simulink model "ARC_DTm"  (R2025b)
settings: Solver=FixedStepAuto  StartTime=0.0  StopTime=10080  FixedStep=1  RelTol=1e-3
PreLoadFcn:
  | %For Preload, set the working path
  | modelFolder = fileparts(which(bdroot));
  | addpath(genpath(modelFolder));
StartFcn:
  | tic
StopFcn:
  | fprintf("Sim Time: %.02f min", toc/60)
values from neighbouring files (symbols this model uses):
  batteryScenario = p.batteryScenario    [RUNSIM_ParameterSweep.m]    (also in _RUNSIM_ParameterSweep.m)
  Electricity_SalePriceModifier = 50/100    (= 0.5)    [RUNSIM_ParameterSweep.m]    (also in _RUNSIM_ParameterSweep.m)
  LUT = LUT_load.gamLUT    [RUNSIM_ParameterSweep.m]    (also in _RUNSIM_ParameterSweep.m)
  minimum_UF_system_flow = 5833    [RUNSIM_ParameterSweep.m]    (also in _RUNSIM_ParameterSweep.m)
  PROS1_recoveryrate = 61    [RUNSIM_ParameterSweep.m]    (also in _RUNSIM_ParameterSweep.m)
  PROS2_recoveryrate = 62    [RUNSIM_ParameterSweep.m]    (also in _RUNSIM_ParameterSweep.m)
  ROstabilization_time = p.ROstabilization_time    [RUNSIM_ParameterSweep.m]    (also in _RUNSIM_ParameterSweep.m)
  solarModifier = maximum_solar_generation / 300    [RUNSIM_ParameterSweep.m]    (also in _RUNSIM_ParameterSweep.m)
  TSRO_recoveryrate = 51    [RUNSIM_ParameterSweep.m]    (also in _RUNSIM_ParameterSweep.m)
  UF_RecoveryRate = 96    [RUNSIM_ParameterSweep.m]    (also in _RUNSIM_ParameterSweep.m)
undefined symbols (not defined in the file or in its folder): A_PROS1, A_PROS2, A_TSRO, B_PROS1, B_PROS2, B_TSRO, BW_Max_Time, BW_Max_Vol_gal, CEB_Max_Time, CEB_Max_Vol_gal, CIP_Max_Time, E, FF, h, L, w
libraries: simulink x40
(part 6 of 11)

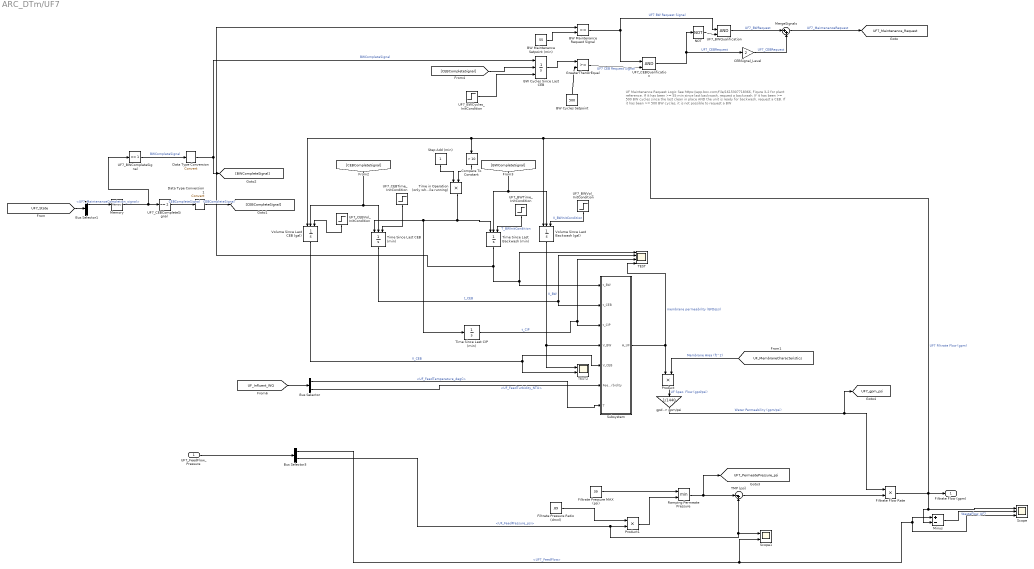
== system ARC_DTm/UF7 ==
  note: UF Maintenance Request Logic
      | See https://app.box.com/file/1615307718366, Figure 3-2 for plant reference.
      |
      | If it has been >= 55 min since last backwash, request a backwash.
      | If it has been >= 500 BW cycles since the last clean in place AND the unit is ready for backwash, request a CEB.
      | If it has been >= 500 BW cycles, it is not possible to request a BW
  UF7_FeedFlow_Pressure : Inport
  BW Cycles Setpoint : Constant  Value=500
  BW Cycles Since Last CEB : Integrator  ExternalReset=rising  InitialConditionSource=external  InitialCondition=5
  BW Maintenance Request Signal : RelationalOperator  OutDataTypeStr=boolean  RndMeth=Simplest  InputSameDT=off
  BW Maintenance Setpoint (min) : Constant  Value=55
  Bus Selector : BusSelector  OutputSignals=UF_FeedTemperature_degC,UF_FeedTurbidity_NTU
  Bus Selector1 : BusSelector  OutputSignals=UF7_MaintenanceCompletion_signal,UF7_OperationsState_signal
  Bus Selector3 : BusSelector  OutputSignals=UF7_FeedFlow,UF_FeedPressure_psi
  CEBSignal_Level : Gain  Gain=2  OutDataTypeStr=double
  Compare To Constant : simulink/Logic and Bit Operations/Compare To Constant  relop=>  const=10  OutDataTypeStr=boolean
  Data Type Conversion : DataTypeConversion  SaturateOnIntegerOverflow=off  RndMeth=Floor
  Data Type Conversion1 : DataTypeConversion  SaturateOnIntegerOverflow=off  RndMeth=Floor
  Filtrate Flow Rate : Product
  Filtrate Pressure MAX (psi) : Constant  Value=39
  Filtrate Pressure Ratio (dmnl) : Constant  Value=.89
  GreaterThanOrEqual : RelationalOperator  OutDataTypeStr=boolean  RndMeth=Simplest  InputSameDT=off
  Memory : Memory
  MergeSignals : Sum  Inputs=|++
  Minus : Sum  Inputs=+-
  NOT : Logic  Operator=NOT  IconShape=distinctive  AllPortsSameDT=off  OutDataTypeStr=boolean
  Product : Product
  Product1 : Product
  Ramping Permeate Pressure : MinMax  Inputs=2
  Scope : Scope  NumInputPorts=3
      settings: ActiveDisplayYMinimum=-126.71796384165732  ActiveDisplayYMaximum=1140.4616745749161  DataLoggingVariableName=ScopeData10
  Scope1 : Scope  NumInputPorts=2
      settings: ActiveDisplayYMinimum=-129.2228584451866  ActiveDisplayYMaximum=1163.0057260066797  DataLoggingVariableName=ScopeData11
  Step Add (min) : Constant
  Subsystem : Subsystem
  TEST : Scope  NumInputPorts=4
      settings: ActiveDisplayYMinimum=13.625  ActiveDisplayYMaximum=27.375  DataLoggingVariableName=ScopeData3
  TEST2 : Scope  NumInputPorts=2
      settings: ActiveDisplayYMinimum=-311929.86683332996  ActiveDisplayYMaximum=2.8073688014999703E+6  DataLoggingVariableName=ScopeData4
  TMP (psi) : Sum  Inputs=|-+
  Time Since Last Backwash (min) : Integrator  ExternalReset=level hold  InitialConditionSource=external  InitialCondition=26
  Time Since Last CEB (min) : Integrator  ExternalReset=level hold  InitialConditionSource=external  InitialCondition=4833
  Time Since Last CIP (min) : Integrator  InitialCondition=round(CIP_Max_Time*rand())
  Time in Operation (only while running) : Product
  UF7_BWCompleteSignal : simulink/Logic and Bit Operations/Compare To Constant  relop===  const=1  OutDataTypeStr=uint8
  UF7_BWCycles_InitCondition : Step  Before=round(500 * rand())  After=0  SampleTime=0
  UF7_BWQualification : Logic  IconShape=distinctive  AllPortsSameDT=off  OutDataTypeStr=boolean
  UF7_BWTime_InitCondition : Step  Before=round(BW_Max_Time*rand())  After=0  SampleTime=0
  UF7_BWVol_InitCondition : Step  Before=round(BW_Max_Vol_gal*rand())  After=0  SampleTime=0
  UF7_CEBCompleteSignal : simulink/Logic and Bit Operations/Compare To Constant  relop===  const=2  OutDataTypeStr=uint8
  UF7_CEBQualification : Logic  IconShape=distinctive  AllPortsSameDT=off  OutDataTypeStr=boolean
  UF7_CEBTime_InitCondition : Step  Before=round(CEB_Max_Time*rand())  After=0  SampleTime=0
  UF7_CEBVol_InitCondition : Step  Before=round(CEB_Max_Vol_gal*rand())  After=0  SampleTime=0
  Volume Since Last Backwash (gal) : Integrator  ExternalReset=level hold  InitialConditionSource=external  InitialCondition=34330
  Volume Since Last CEB (gal) : Integrator  ExternalReset=rising  InitialConditionSource=external  InitialCondition=2777254
  "gpd -> gpm/psi" : Gain  Gain=1/1440
  Filtrate Flow (gpm) : Outport
  tag scope: UF7_Maintenance_Request=global, UF7_PermeatePressure_psi=global, UF7_gpm_psi=global
  wires:
  Volume Since Last Backwash (gal)/1 -> Subsystem/4(V_BW), TEST2/1  "V_BW"
  Time Since Last Backwash (min)/1 -> BW Maintenance Request Signal/1, Subsystem/1(t_BW), TEST/1
  Product/1 -> "gpd -> gpm/psi"/1  "UF Spec. Flow (gpd/psi)"
  [UF_MembraneCharacteristics] -> Product/2  "Membrane Area (ft^2)"
  "gpd -> gpm/psi"/1 -> Filtrate Flow Rate/1, [UF7_gpm_psi]  "Water Permeability (gpm/psi)"
  Time in Operation (only while running)/1 -> Time Since Last Backwash (min)/1, Time Since Last CEB (min)/1, Time Since Last CIP (min)/1
  Filtrate Flow Rate/1 -> Scope/1, Minus/2, Volume Since Last Backwash (gal)/1, Volume Since Last CEB (gal)/1, Compare To Constant/1, Filtrate Flow (gpm)/1  "UF7 Filtrate Flow (gpm)"
  Time Since Last CEB (min)/1 -> Subsystem/2(t_CEB), TEST/2  "t_CEB"
  Volume Since Last CEB (gal)/1 -> Subsystem/5(V_CEB), TEST2/2  "V_CEB"
  Time Since Last CIP (min)/1 -> Subsystem/3(t_CIP), TEST/3  "t_CIP"
  Filtrate Pressure MAX (psi)/1 -> Ramping Permeate Pressure/1
  [UF_Influent_WQ] -> Bus Selector/1
  Bus Selector/1 -> Subsystem/7(T)  "<UF_FeedTemperature_degC>"
  UF7_FeedFlow_Pressure/1 -> Bus Selector3/1
  Filtrate Pressure Ratio (dmnl)/1 -> Product1/1
  Product1/1 -> Ramping Permeate Pressure/2
  Ramping Permeate Pressure/1 -> [UF7_PermeatePressure_psi], TMP (psi)/1
  TMP (psi)/1 -> Filtrate Flow Rate/2
  BW Maintenance Setpoint (min)/1 -> BW Maintenance Request Signal/2
  BW Cycles Since Last CEB/1 -> GreaterThanOrEqual/1
  BW Cycles Setpoint/1 -> GreaterThanOrEqual/2
  Bus Selector/2 -> Subsystem/6(Feed Turbidity)  "<UF_FeedTurbidity_NTU>"
  [UF7_State] -> Bus Selector1/1
  MergeSignals/1 -> [UF7_Maintenance_Request]  "UF7_MaintenanceRequest"
  UF7_CEBCompleteSignal/1 -> Data Type Conversion1/1  "CEBCompleteSignal"
  [CEBCompleteSignal] -> Volume Since Last CEB (gal)/2, Time Since Last CEB (min)/2
  Data Type Conversion/1 -> [BWCompleteSignal], BW Cycles Since Last CEB/1  "BWCompleteSignal"
  [BWCompleteSignal] -> Volume Since Last Backwash (gal)/2, Time Since Last Backwash (min)/2
  [CEBCompleteSignal] -> BW Cycles Since Last CEB/2
  Bus Selector1/1 -> Memory/1  "<UF7_MaintenanceCompletion_signal>"
  UF7_BWCompleteSignal/1 -> Data Type Conversion/1  "BWCompleteSignal"
  Data Type Conversion1/1 -> [CEBCompleteSignal]  "CEBCompleteSignal"
  UF7_BWCycles_InitCondition/1 -> BW Cycles Since Last CEB/3
  Subsystem/1(A_UF) -> TEST/4, Product/1  "membrane permeability (GFD/psi)"
  UF7_BWTime_InitCondition/1 -> Time Since Last Backwash (min)/3  "T_BWInitCondition"
  UF7_CEBVol_InitCondition/1 -> Volume Since Last CEB (gal)/3
  UF7_CEBTime_InitCondition/1 -> Time Since Last CEB (min)/3
  UF7_BWVol_InitCondition/1 -> Volume Since Last Backwash (gal)/3  "V_BWInitCondition"
  Step Add (min)/1 -> Time in Operation (only while running)/1
  Compare To Constant/1 -> Time in Operation (only while running)/2
  Memory/1 -> UF7_BWCompleteSignal/1, UF7_CEBCompleteSignal/1
  UF7_BWQualification/1 -> MergeSignals/1  "UF7_BWRequest"
  GreaterThanOrEqual/1 -> UF7_CEBQualification/2  "UF7 CEB Request Signal"
  UF7_CEBQualification/1 -> CEBSignal_Level/1, NOT/1  "UF7_CEBRequest"
  BW Maintenance Request Signal/1 -> UF7_BWQualification/1, UF7_CEBQualification/1  "UF7 BW Request Signal"
  NOT/1 -> UF7_BWQualification/2
  CEBSignal_Level/1 -> MergeSignals/2  "UF7_CEBRequest"
  Bus Selector3/1 -> Scope1/2, Minus/1, Scope/3  "<UF7_FeedFlow>"
  Bus Selector3/2 -> TMP (psi)/2, Scope1/1, Product1/2  "<UF_FeedPressure_psi>"
  Minus/1 -> Scope/2  "WasteFlow_UF7"

== system ARC_DTm/UF8 ==
  note: UF Maintenance Request Logic
      | See https://app.box.com/file/1615307718366, Figure 3-2 for plant reference.
      |
      | If it has been >= 55 min since last backwash, request a backwash.
      | If it has been >= 500 BW cycles since the last clean in place AND the unit is ready for backwash, request a CEB.
      | If it has been >= 500 BW cycles, it is not possible to request a BW
  UF8_FeedFlow_Pressure : Inport
  BW Cycles Setpoint : Constant  Value=500
  BW Cycles Since Last CEB : Integrator  ExternalReset=rising  InitialConditionSource=external  InitialCondition=5
  BW Maintenance Request Signal : RelationalOperator  OutDataTypeStr=boolean  RndMeth=Simplest  InputSameDT=off
  BW Maintenance Setpoint (min) : Constant  Value=55
  Bus Selector : BusSelector  OutputSignals=UF_FeedTemperature_degC,UF_FeedTurbidity_NTU
  Bus Selector1 : BusSelector  OutputSignals=UF8_MaintenanceCompletion_signal,UF8_OperationsState_signal
  Bus Selector3 : BusSelector  OutputSignals=UF8_FeedFlow,UF_FeedPressure_psi
  CEBSignal_Level : Gain  Gain=2  OutDataTypeStr=double
  Compare To Constant : simulink/Logic and Bit Operations/Compare To Constant  relop=>  const=10  OutDataTypeStr=boolean
  Data Type Conversion : DataTypeConversion  SaturateOnIntegerOverflow=off  RndMeth=Floor
  Data Type Conversion1 : DataTypeConversion  SaturateOnIntegerOverflow=off  RndMeth=Floor
  Filtrate Flow Rate : Product
  Filtrate Pressure MAX (psi) : Constant  Value=39
  Filtrate Pressure Ratio (dmnl) : Constant  Value=.89
  GreaterThanOrEqual : RelationalOperator  OutDataTypeStr=boolean  RndMeth=Simplest  InputSameDT=off
  Memory : Memory
  MergeSignals : Sum  Inputs=|++
  Minus : Sum  Inputs=+-
  NOT : Logic  Operator=NOT  IconShape=distinctive  AllPortsSameDT=off  OutDataTypeStr=boolean
  Product : Product
  Product1 : Product
  Ramping Permeate Pressure : MinMax  Inputs=2
  Scope : Scope  NumInputPorts=3
      settings: ActiveDisplayYMinimum=-126.71796384165732  ActiveDisplayYMaximum=1140.4616745749161  DataLoggingVariableName=ScopeData10
  Scope1 : Scope  NumInputPorts=2
      settings: ActiveDisplayYMinimum=-129.2228584451866  ActiveDisplayYMaximum=1163.0057260066797  DataLoggingVariableName=ScopeData11
  Step Add (min) : Constant
  Subsystem : Subsystem
  TEST : Scope  NumInputPorts=4
      settings: ActiveDisplayYMinimum=13.625  ActiveDisplayYMaximum=27.375  DataLoggingVariableName=ScopeData3
  TEST2 : Scope  NumInputPorts=2
      settings: ActiveDisplayYMinimum=-311929.86683332996  ActiveDisplayYMaximum=2.8073688014999703E+6  DataLoggingVariableName=ScopeData4
  TMP (psi) : Sum  Inputs=|-+
  Time Since Last Backwash (min) : Integrator  ExternalReset=level hold  InitialConditionSource=external  InitialCondition=26
  Time Since Last CEB (min) : Integrator  ExternalReset=level hold  InitialConditionSource=external  InitialCondition=4833
  Time Since Last CIP (min) : Integrator  InitialCondition=round(CIP_Max_Time*rand())
  Time in Operation (only while running) : Product
  UF8_BWCompleteSignal : simulink/Logic and Bit Operations/Compare To Constant  relop===  const=1  OutDataTypeStr=uint8
  UF8_BWCycles_InitCondition : Step  Before=round(500 * rand())  After=0  SampleTime=0
  UF8_BWQualification : Logic  IconShape=distinctive  AllPortsSameDT=off  OutDataTypeStr=boolean
  UF8_BWTime_InitCondition : Step  Before=round(BW_Max_Time*rand())  After=0  SampleTime=0
  UF8_BWVol_InitCondition : Step  Before=round(BW_Max_Vol_gal*rand())  After=0  SampleTime=0
  UF8_CEBCompleteSignal : simulink/Logic and Bit Operations/Compare To Constant  relop===  const=2  OutDataTypeStr=uint8
  UF8_CEBQualification : Logic  IconShape=distinctive  AllPortsSameDT=off  OutDataTypeStr=boolean
  UF8_CEBTime_InitCondition : Step  Before=round(CEB_Max_Time*rand())  After=0  SampleTime=0
  UF8_CEBVol_InitCondition : Step  Before=round(CEB_Max_Vol_gal*rand())  After=0  SampleTime=0
  Volume Since Last Backwash (gal) : Integrator  ExternalReset=level hold  InitialConditionSource=external  InitialCondition=34330
  Volume Since Last CEB (gal) : Integrator  ExternalReset=rising  InitialConditionSource=external  InitialCondition=2777254
  "gpd -> gpm/psi" : Gain  Gain=1/1440
  Filtrate Flow (gpm) : Outport
  tag scope: UF8_Maintenance_Request=global, UF8_PermeatePressure_psi=global, UF8_gpm_psi=global
  wires:
  Volume Since Last Backwash (gal)/1 -> Subsystem/4(V_BW), TEST2/1  "V_BW"
  Time Since Last Backwash (min)/1 -> BW Maintenance Request Signal/1, Subsystem/1(t_BW), TEST/1
  Product/1 -> "gpd -> gpm/psi"/1  "UF Spec. Flow (gpd/psi)"
  [UF_MembraneCharacteristics] -> Product/2  "Membrane Area (ft^2)"
  "gpd -> gpm/psi"/1 -> Filtrate Flow Rate/1, [UF8_gpm_psi]  "Water Permeability (gpm/psi)"
  Time in Operation (only while running)/1 -> Time Since Last Backwash (min)/1, Time Since Last CEB (min)/1, Time Since Last CIP (min)/1
  Filtrate Flow Rate/1 -> Scope/1, Minus/2, Volume Since Last Backwash (gal)/1, Volume Since Last CEB (gal)/1, Compare To Constant/1, Filtrate Flow (gpm)/1  "UF8 Filtrate Flow (gpm)"
  Time Since Last CEB (min)/1 -> Subsystem/2(t_CEB), TEST/2  "t_CEB"
  Volume Since Last CEB (gal)/1 -> Subsystem/5(V_CEB), TEST2/2  "V_CEB"
  Time Since Last CIP (min)/1 -> Subsystem/3(t_CIP), TEST/3  "t_CIP"
  Filtrate Pressure MAX (psi)/1 -> Ramping Permeate Pressure/1
  [UF_Influent_WQ] -> Bus Selector/1
  Bus Selector/1 -> Subsystem/7(T)  "<UF_FeedTemperature_degC>"
  UF8_FeedFlow_Pressure/1 -> Bus Selector3/1
  Filtrate Pressure Ratio (dmnl)/1 -> Product1/1
  Product1/1 -> Ramping Permeate Pressure/2
  Ramping Permeate Pressure/1 -> [UF8_PermeatePressure_psi], TMP (psi)/1
  TMP (psi)/1 -> Filtrate Flow Rate/2
  BW Maintenance Setpoint (min)/1 -> BW Maintenance Request Signal/2
  BW Cycles Since Last CEB/1 -> GreaterThanOrEqual/1
  BW Cycles Setpoint/1 -> GreaterThanOrEqual/2
  Bus Selector/2 -> Subsystem/6(Feed Turbidity)  "<UF_FeedTurbidity_NTU>"
  [UF8_State] -> Bus Selector1/1
  MergeSignals/1 -> [UF8_Maintenance_Request]  "UF8_MaintenanceRequest"
  UF8_CEBCompleteSignal/1 -> Data Type Conversion1/1  "CEBCompleteSignal"
  [CEBCompleteSignal] -> Volume Since Last CEB (gal)/2, Time Since Last CEB (min)/2
  Data Type Conversion/1 -> [BWCompleteSignal], BW Cycles Since Last CEB/1  "BWCompleteSignal"
  [BWCompleteSignal] -> Volume Since Last Backwash (gal)/2, Time Since Last Backwash (min)/2
  [CEBCompleteSignal] -> BW Cycles Since Last CEB/2
  Bus Selector1/1 -> Memory/1  "<UF8_MaintenanceCompletion_signal>"
  UF8_BWCompleteSignal/1 -> Data Type Conversion/1  "BWCompleteSignal"
  Data Type Conversion1/1 -> [CEBCompleteSignal]  "CEBCompleteSignal"
  UF8_BWCycles_InitCondition/1 -> BW Cycles Since Last CEB/3
  Subsystem/1(A_UF) -> TEST/4, Product/1  "membrane permeability (GFD/psi)"
  UF8_BWTime_InitCondition/1 -> Time Since Last Backwash (min)/3  "T_BWInitCondition"
  UF8_CEBVol_InitCondition/1 -> Volume Since Last CEB (gal)/3
  UF8_CEBTime_InitCondition/1 -> Time Since Last CEB (min)/3
  UF8_BWVol_InitCondition/1 -> Volume Since Last Backwash (gal)/3  "V_BWInitCondition"
  Step Add (min)/1 -> Time in Operation (only while running)/1
  Compare To Constant/1 -> Time in Operation (only while running)/2
  Memory/1 -> UF8_BWCompleteSignal/1, UF8_CEBCompleteSignal/1
  UF8_BWQualification/1 -> MergeSignals/1  "UF8_BWRequest"
  GreaterThanOrEqual/1 -> UF8_CEBQualification/2  "UF8 CEB Request Signal"
  UF8_CEBQualification/1 -> CEBSignal_Level/1, NOT/1  "UF8_CEBRequest"
  BW Maintenance Request Signal/1 -> UF8_BWQualification/1, UF8_CEBQualification/1  "UF8 BW Request Signal"
  NOT/1 -> UF8_BWQualification/2
  CEBSignal_Level/1 -> MergeSignals/2  "UF8_CEBRequest"
  Bus Selector3/1 -> Scope1/2, Minus/1, Scope/3  "<UF8_FeedFlow>"
  Bus Selector3/2 -> TMP (psi)/2, Scope1/1, Product1/2  "<UF_FeedPressure_psi>"
  Minus/1 -> Scope/2  "WasteFlow_UF8"

== system ARC_DTm/UF9 ==
  note: UF Maintenance Request Logic
      | See https://app.box.com/file/1615307718366, Figure 3-2 for plant reference.
      |
      | If it has been >= 55 min since last backwash, request a backwash.
      | If it has been >= 500 BW cycles since the last clean in place AND the unit is ready for backwash, request a CEB.
      | If it has been >= 500 BW cycles, it is not possible to request a BW
  UF9_FeedFlow_Pressure : Inport
  BW Cycles Setpoint : Constant  Value=500
  BW Cycles Since Last CEB : Integrator  ExternalReset=rising  InitialConditionSource=external  InitialCondition=5
  BW Maintenance Request Signal : RelationalOperator  OutDataTypeStr=boolean  RndMeth=Simplest  InputSameDT=off
  BW Maintenance Setpoint (min) : Constant  Value=55
  Bus Selector : BusSelector  OutputSignals=UF_FeedTemperature_degC,UF_FeedTurbidity_NTU
  Bus Selector1 : BusSelector  OutputSignals=UF9_MaintenanceCompletion_signal,UF9_OperationsState_signal
  Bus Selector3 : BusSelector  OutputSignals=UF9_FeedFlow,UF_FeedPressure_psi
  CEBSignal_Level : Gain  Gain=2  OutDataTypeStr=double
  Compare To Constant : simulink/Logic and Bit Operations/Compare To Constant  relop=>  const=10  OutDataTypeStr=boolean
  Data Type Conversion : DataTypeConversion  SaturateOnIntegerOverflow=off  RndMeth=Floor
  Data Type Conversion1 : DataTypeConversion  SaturateOnIntegerOverflow=off  RndMeth=Floor
  Filtrate Flow Rate : Product
  Filtrate Pressure MAX (psi) : Constant  Value=39
  Filtrate Pressure Ratio (dmnl) : Constant  Value=.89
  GreaterThanOrEqual : RelationalOperator  OutDataTypeStr=boolean  RndMeth=Simplest  InputSameDT=off
  Memory : Memory
  MergeSignals : Sum  Inputs=|++
  Minus : Sum  Inputs=+-
  NOT : Logic  Operator=NOT  IconShape=distinctive  AllPortsSameDT=off  OutDataTypeStr=boolean
  Product : Product
  Product1 : Product
  Ramping Permeate Pressure : MinMax  Inputs=2
  Scope : Scope  NumInputPorts=3
      settings: ActiveDisplayYMinimum=-126.71796384165732  ActiveDisplayYMaximum=1140.4616745749161  DataLoggingVariableName=ScopeData10
  Scope1 : Scope  NumInputPorts=2
      settings: ActiveDisplayYMinimum=-129.2228584451866  ActiveDisplayYMaximum=1163.0057260066797  DataLoggingVariableName=ScopeData11
  Step Add (min) : Constant
  Subsystem : Subsystem
  TEST : Scope  NumInputPorts=4
      settings: ActiveDisplayYMinimum=13.625  ActiveDisplayYMaximum=27.375  DataLoggingVariableName=ScopeData3
  TEST2 : Scope  NumInputPorts=2
      settings: ActiveDisplayYMinimum=-311929.86683332996  ActiveDisplayYMaximum=2.8073688014999703E+6  DataLoggingVariableName=ScopeData4
  TMP (psi) : Sum  Inputs=|-+
  Time Since Last Backwash (min) : Integrator  ExternalReset=level hold  InitialConditionSource=external  InitialCondition=26
  Time Since Last CEB (min) : Integrator  ExternalReset=level hold  InitialConditionSource=external  InitialCondition=4833
  Time Since Last CIP (min) : Integrator  InitialCondition=round(CIP_Max_Time*rand())
  Time in Operation (only while running) : Product
  UF9_BWCompleteSignal : simulink/Logic and Bit Operations/Compare To Constant  relop===  const=1  OutDataTypeStr=uint8
  UF9_BWCycles_InitCondition : Step  Before=round(500 * rand())  After=0  SampleTime=0
  UF9_BWQualification : Logic  IconShape=distinctive  AllPortsSameDT=off  OutDataTypeStr=boolean
  UF9_BWTime_InitCondition : Step  Before=round(BW_Max_Time*rand())  After=0  SampleTime=0
  UF9_BWVol_InitCondition : Step  Before=round(BW_Max_Vol_gal*rand())  After=0  SampleTime=0
  UF9_CEBCompleteSignal : simulink/Logic and Bit Operations/Compare To Constant  relop===  const=2  OutDataTypeStr=uint8
  UF9_CEBQualification : Logic  IconShape=distinctive  AllPortsSameDT=off  OutDataTypeStr=boolean
  UF9_CEBTime_InitCondition : Step  Before=round(CEB_Max_Time*rand())  After=0  SampleTime=0
  UF9_CEBVol_InitCondition : Step  Before=round(CEB_Max_Vol_gal*rand())  After=0  SampleTime=0
  Volume Since Last Backwash (gal) : Integrator  ExternalReset=level hold  InitialConditionSource=external  InitialCondition=34330
  Volume Since Last CEB (gal) : Integrator  ExternalReset=rising  InitialConditionSource=external  InitialCondition=2777254
  "gpd -> gpm/psi" : Gain  Gain=1/1440
  Filtrate Flow (gpm) : Outport
  tag scope: UF9_Maintenance_Request=global, UF9_PermeatePressure_psi=global, UF9_gpm_psi=global
  wires:
  Volume Since Last Backwash (gal)/1 -> Subsystem/4(V_BW), TEST2/1  "V_BW"
  Time Since Last Backwash (min)/1 -> BW Maintenance Request Signal/1, Subsystem/1(t_BW), TEST/1
  Product/1 -> "gpd -> gpm/psi"/1  "UF Spec. Flow (gpd/psi)"
  [UF_MembraneCharacteristics] -> Product/2  "Membrane Area (ft^2)"
  "gpd -> gpm/psi"/1 -> Filtrate Flow Rate/1, [UF9_gpm_psi]  "Water Permeability (gpm/psi)"
  Time in Operation (only while running)/1 -> Time Since Last Backwash (min)/1, Time Since Last CEB (min)/1, Time Since Last CIP (min)/1
  Filtrate Flow Rate/1 -> Scope/1, Minus/2, Volume Since Last Backwash (gal)/1, Volume Since Last CEB (gal)/1, Compare To Constant/1, Filtrate Flow (gpm)/1  "UF9 Filtrate Flow (gpm)"
  Time Since Last CEB (min)/1 -> Subsystem/2(t_CEB), TEST/2  "t_CEB"
  Volume Since Last CEB (gal)/1 -> Subsystem/5(V_CEB), TEST2/2  "V_CEB"
  Time Since Last CIP (min)/1 -> Subsystem/3(t_CIP), TEST/3  "t_CIP"
  Filtrate Pressure MAX (psi)/1 -> Ramping Permeate Pressure/1
  [UF_Influent_WQ] -> Bus Selector/1
  Bus Selector/1 -> Subsystem/7(T)  "<UF_FeedTemperature_degC>"
  UF9_FeedFlow_Pressure/1 -> Bus Selector3/1
  Filtrate Pressure Ratio (dmnl)/1 -> Product1/1
  Product1/1 -> Ramping Permeate Pressure/2
  Ramping Permeate Pressure/1 -> [UF9_PermeatePressure_psi], TMP (psi)/1
  TMP (psi)/1 -> Filtrate Flow Rate/2
  BW Maintenance Setpoint (min)/1 -> BW Maintenance Request Signal/2
  BW Cycles Since Last CEB/1 -> GreaterThanOrEqual/1
  BW Cycles Setpoint/1 -> GreaterThanOrEqual/2
  Bus Selector/2 -> Subsystem/6(Feed Turbidity)  "<UF_FeedTurbidity_NTU>"
  [UF9_State] -> Bus Selector1/1
  MergeSignals/1 -> [UF9_Maintenance_Request]  "UF9_MaintenanceRequest"
  UF9_CEBCompleteSignal/1 -> Data Type Conversion1/1  "CEBCompleteSignal"
  [CEBCompleteSignal] -> Volume Since Last CEB (gal)/2, Time Since Last CEB (min)/2
  Data Type Conversion/1 -> [BWCompleteSignal], BW Cycles Since Last CEB/1  "BWCompleteSignal"
  [BWCompleteSignal] -> Volume Since Last Backwash (gal)/2, Time Since Last Backwash (min)/2
  [CEBCompleteSignal] -> BW Cycles Since Last CEB/2
  Bus Selector1/1 -> Memory/1  "<UF9_MaintenanceCompletion_signal>"
  UF9_BWCompleteSignal/1 -> Data Type Conversion/1  "BWCompleteSignal"
  Data Type Conversion1/1 -> [CEBCompleteSignal]  "CEBCompleteSignal"
  UF9_BWCycles_InitCondition/1 -> BW Cycles Since Last CEB/3
  Subsystem/1(A_UF) -> TEST/4, Product/1  "membrane permeability (GFD/psi)"
  UF9_BWTime_InitCondition/1 -> Time Since Last Backwash (min)/3  "T_BWInitCondition"
  UF9_CEBVol_InitCondition/1 -> Volume Since Last CEB (gal)/3
  UF9_CEBTime_InitCondition/1 -> Time Since Last CEB (min)/3
  UF9_BWVol_InitCondition/1 -> Volume Since Last Backwash (gal)/3  "V_BWInitCondition"
  Step Add (min)/1 -> Time in Operation (only while running)/1
  Compare To Constant/1 -> Time in Operation (only while running)/2
  Memory/1 -> UF9_BWCompleteSignal/1, UF9_CEBCompleteSignal/1
  UF9_BWQualification/1 -> MergeSignals/1  "UF9_BWRequest"
  GreaterThanOrEqual/1 -> UF9_CEBQualification/2  "UF9 CEB Request Signal"
  UF9_CEBQualification/1 -> CEBSignal_Level/1, NOT/1  "UF9_CEBRequest"
  BW Maintenance Request Signal/1 -> UF9_BWQualification/1, UF9_CEBQualification/1  "UF9 BW Request Signal"
  NOT/1 -> UF9_BWQualification/2
  CEBSignal_Level/1 -> MergeSignals/2  "UF9_CEBRequest"
  Bus Selector3/1 -> Scope1/2, Minus/1, Scope/3  "<UF9_FeedFlow>"
  Bus Selector3/2 -> TMP (psi)/2, Scope1/1, Product1/2  "<UF_FeedPressure_psi>"
  Minus/1 -> Scope/2  "WasteFlow_UF9"

== system ARC_DTm/UF_Feed_Manifold ==
  UF_Pump_Discharge : Inport
  Bus Creator{,1..10} (11 alike) : BusCreator  Inputs=2
  Bus Selector : BusSelector  OutputSignals=UFFeedFlow_Setpoint_gpm,UFFeedFlow_Actual_gpm
  Demux : Demux  Outputs=10
  Demux1 : Demux  Outputs=10
  MATLAB Function : MATLAB Function  TreatAsAtomicUnit=on
  Memory3 : Memory
  Mux1 : Mux  Inputs=10
  Mux2 : Mux  Inputs=10
  Scope : Scope  NumInputPorts=2
      settings: ActiveDisplayYMinimum=5507.4375  ActiveDisplayYMaximum=8763.0625  DataLoggingVariableName=ScopeData34
  Scope4 : Scope
      settings: ActiveDisplayYMinimum=-192.8571428571428  ActiveDisplayYMaximum=1735.7142857142858  DataLoggingVariableName=ScopeData38
  UF Flow Maximum (gpm) : Constant  Value=1640
  UF_Dispatcher : MATLAB Function  TreatAsAtomicUnit=on
  To UF1 : Outport
  To UF2 : Outport  Port=2
  To UF3 : Outport  Port=3
  To UF4 : Outport  Port=4
  To UF5 : Outport  Port=5
  To UF6 : Outport  Port=6
  To UF7 : Outport  Port=7
  To UF8 : Outport  Port=8
  To UF9 : Outport  Port=9
  To UF10 : Outport  Port=10
  tag scope: UFMembrane_FlowVector=global, UFPump_FeedPressure_psi=global, UF_Influent_WQ=global
  wires:
  Bus Creator5/1 -> To UF5/1
  Bus Creator2/1 -> To UF2/1
  Demux/6 -> Bus Creator6/1  "UF6_FeedFlow"
  Demux/3 -> Bus Creator3/1  "UF3_FeedFlow"
  [UF4_gpm_psi] -> Mux1/4
  [UF2_gpm_psi] -> Mux1/2
  [UF1_gpm_psi] -> Mux1/1
  [UF10_PermeatePressure_psi] -> Mux2/10
  [UF3_gpm_psi] -> Mux1/3
  [UF4_PermeatePressure_psi] -> Mux2/4
  [UF5_gpm_psi] -> Mux1/5
  [UF6_gpm_psi] -> Mux1/6
  [UF3_PermeatePressure_psi] -> Mux2/3
  [UF7_gpm_psi] -> Mux1/7
  [UF5_PermeatePressure_psi] -> Mux2/5
  [UF8_gpm_psi] -> Mux1/8
  [UF9_gpm_psi] -> Mux1/9
  [UF10_gpm_psi] -> Mux1/10
  Bus Creator3/1 -> To UF3/1
  [UF1_PermeatePressure_psi] -> Mux2/1
  Demux1/3 -> Bus Creator3/2  "UF_FeedPressure_psi"
  [UF2_PermeatePressure_psi] -> Mux2/2
  Bus Creator4/1 -> To UF4/1
  Demux1/5 -> Bus Creator5/2  "UF_FeedPressure_psi"
  [UF6_PermeatePressure_psi] -> Mux2/6
  [UF7_PermeatePressure_psi] -> Mux2/7
  UF_Dispatcher/1(flows) -> [UFMembrane_FlowVector], Demux/1, MATLAB Function/1(prescribed_feedflow_vec), Scope4/1, Memory3/1
  [UF8_PermeatePressure_psi] -> Mux2/8
  [UF9_PermeatePressure_psi] -> Mux2/9
  Bus Creator/1 -> [UF_Influent_WQ]
  Demux1/4 -> Bus Creator4/2  "UF_FeedPressure_psi"
  Demux/4 -> Bus Creator4/1  "UF4_FeedFlow"
  Mux1/1 -> MATLAB Function/2(membrane_conductance_vec)
  Mux2/1 -> MATLAB Function/3(UF_PermeatePressure_vec)  "psi"
  MATLAB Function/1(UF_FeedPressure_vector) -> Demux1/1
  MATLAB Function/2(UFPump_Pressure_Setpoint) -> [UFPump_FeedPressure_psi]
  Demux/1 -> Bus Creator1/1  "UF1_FeedFlow"
  Bus Creator1/1 -> To UF1/1
  Demux/2 -> Bus Creator2/1  "UF2_FeedFlow"
  Demux/5 -> Bus Creator5/1  "UF5_FeedFlow"
  Demux1/1 -> Bus Creator1/2  "UF_FeedPressure_psi"
  Demux1/2 -> Bus Creator2/2  "UF_FeedPressure_psi"
  Demux1/6 -> Bus Creator6/2  "UF_FeedPressure_psi"
  Bus Creator6/1 -> To UF6/1
  Bus Creator7/1 -> To UF7/1
  Demux1/7 -> Bus Creator7/2  "UF_FeedPressure_psi"
  Demux/7 -> Bus Creator7/1  "UF7_FeedFlow"
  Bus Creator8/1 -> To UF8/1
  Demux1/8 -> Bus Creator8/2  "UF_FeedPressure_psi"
  Demux/8 -> Bus Creator8/1  "UF8_FeedFlow"
  Bus Creator9/1 -> To UF9/1
  Demux1/9 -> Bus Creator9/2  "UF_FeedPressure_psi"
  Demux/9 -> Bus Creator9/1  "UF9_FeedFlow"
  Bus Creator10/1 -> To UF10/1
  Demux1/10 -> Bus Creator10/2  "UF_FeedPressure_psi"
  Demux/10 -> Bus Creator10/1  "UF10_FeedFlow"
  [FeedTurbidity_NTU] -> Bus Creator/2  "UF_FeedTurbidity_NTU"
  [T] -> Bus Creator/1  "UF_FeedTemperature_degC"
  UF Flow Maximum (gpm)/1 -> UF_Dispatcher/1(max_flow_per_unit)
  Bus Selector/2 -> Scope/1, UF_Dispatcher/2(flow_actual)  "<UFFeedFlow_Actual_gpm>"
  Memory3/1 -> UF_Dispatcher/4(prev_flows)
  UF_Pump_Discharge/1 -> Bus Selector/1
  Bus Selector/1 -> Scope/2, UF_Dispatcher/3(flow_setpoint)  "<UFFeedFlow_Setpoint_gpm>"

== system ARC_DTm/UVAOP 1 ==
  feedFlow_gpm : Inport
  Constant : Constant  Value=0
  MATLAB Function : MATLAB Function  TreatAsAtomicUnit=on
  Switch : Switch  Criteria=u2 > Threshold  SaturateOnIntegerOverflow=off  InputSameDT=off
  powerKW : Outport
  tag scope: UVAOP_1_kW=global
  wires:
  feedFlow_gpm/1 -> Switch/2, MATLAB Function/1(feedFlow_gpm)
  Switch/1 -> powerKW/1, [UVAOP_1_kW]
  MATLAB Function/1(powerKW) -> Switch/1
  Constant/1 -> Switch/3

== system ARC_DTm/UVAOP 2 ==
  feedFlow_gpm : Inport
  Constant : Constant  Value=0
  Display : Display
  MATLAB Function : MATLAB Function  TreatAsAtomicUnit=on
  Switch : Switch  Criteria=u2 > Threshold  SaturateOnIntegerOverflow=off  InputSameDT=off
  powerKW : Outport
  tag scope: UVAOP_2_kW=global
  wires:
  feedFlow_gpm/1 -> MATLAB Function/1(feedFlow_gpm), Switch/2
  Switch/1 -> Display/1, [UVAOP_2_kW], powerKW/1
  Constant/1 -> Switch/3
  MATLAB Function/1(powerKW) -> Switch/1

== system ARC_DTm/PROS1_1/Subsystem ==
  <Feed Temperature (oC)> : Inport
  <S1 Feed Pressure (bar)> : Inport  Port=2
  Pperm : Inport  Port=3
  Water Perm (L/m2/min/Bar) : Inport  Port=4
  Salt Perm (L/m2/min) : Inport  Port=5
  <S1 Feed Salinity (g/L)> : Inport  Port=6
  cperm : Inport  Port=7
  Jw : Inport  Port=8
  dh : Inport  Port=9
  L : Inport  Port=10
  u : Inport  Port=11
  MATLAB Function : MATLAB Function  TreatAsAtomicUnit=on
  Permeate Flux Rate (L/min/m2) : Outport
  Permeate Salinity g/L : Outport  Port=2
  deltaPi_bar : Outport  Port=3
  wires:
  Salt Perm (L/m2/min)/1 -> MATLAB Function/5(B)
  <Feed Temperature (oC)>/1 -> MATLAB Function/1(T)
  <S1 Feed Salinity (g/L)>/1 -> MATLAB Function/6(cfeed)
  <S1 Feed Pressure (bar)>/1 -> MATLAB Function/2(Pfeed)
  cperm/1 -> MATLAB Function/7(cperm_prev)
  Pperm/1 -> MATLAB Function/3(Pperm)
  Jw/1 -> MATLAB Function/8(Jw_prev)
  Water Perm (L/m2/min/Bar)/1 -> MATLAB Function/4(A)
  dh/1 -> MATLAB Function/9(dh)
  L/1 -> MATLAB Function/10(L)
  u/1 -> MATLAB Function/11(u)
  MATLAB Function/1(Jw) -> Permeate Flux Rate (L/min/m2)/1  "Permeate Flux Rate (L/min/m2)"
  MATLAB Function/2(cperm) -> Permeate Salinity g/L/1  "PROS1_1_PermeateSalinity_gL"
  MATLAB Function/3(deltaPi_bar) -> deltaPi_bar/1

== system ARC_DTm/PROS1_2/Subsystem ==
  <Feed Temperature (oC)> : Inport
  <S1 Feed Pressure (bar)> : Inport  Port=2
  Pperm : Inport  Port=3
  Water Perm (L/m2/min/Bar) : Inport  Port=4
  Salt Perm (L/m2/min) : Inport  Port=5
  <S1 Feed Salinity (g/L)> : Inport  Port=6
  cperm : Inport  Port=7
  Jw : Inport  Port=8
  dh : Inport  Port=9
  L : Inport  Port=10
  u : Inport  Port=11
  MATLAB Function : MATLAB Function  TreatAsAtomicUnit=on
  Permeate Flux Rate (L/min/m2) : Outport
  Permeate Salinity g/L : Outport  Port=2
  deltaPi_bar : Outport  Port=3
  wires:
  Salt Perm (L/m2/min)/1 -> MATLAB Function/5(B)
  <Feed Temperature (oC)>/1 -> MATLAB Function/1(T)
  <S1 Feed Salinity (g/L)>/1 -> MATLAB Function/6(cfeed)
  <S1 Feed Pressure (bar)>/1 -> MATLAB Function/2(Pfeed)
  cperm/1 -> MATLAB Function/7(cperm_prev)
  Pperm/1 -> MATLAB Function/3(Pperm)
  Jw/1 -> MATLAB Function/8(Jw_prev)
  Water Perm (L/m2/min/Bar)/1 -> MATLAB Function/4(A)
  dh/1 -> MATLAB Function/9(dh)
  L/1 -> MATLAB Function/10(L)
  u/1 -> MATLAB Function/11(u)
  MATLAB Function/1(Jw) -> Permeate Flux Rate (L/min/m2)/1  "Permeate Flux Rate (L/min/m2)"
  MATLAB Function/2(cperm) -> Permeate Salinity g/L/1  "PROS1_2_PermeateSalinity_gL"
  MATLAB Function/3(deltaPi_bar) -> deltaPi_bar/1

== system ARC_DTm/PROS1_3/Subsystem ==
  <Feed Temperature (oC)> : Inport
  <S1 Feed Pressure (bar)> : Inport  Port=2
  Pperm : Inport  Port=3
  Water Perm (L/m2/min/Bar) : Inport  Port=4
  Salt Perm (L/m2/min) : Inport  Port=5
  <S1 Feed Salinity (g/L)> : Inport  Port=6
  cperm : Inport  Port=7
  Jw : Inport  Port=8
  dh : Inport  Port=9
  L : Inport  Port=10
  u : Inport  Port=11
  MATLAB Function : MATLAB Function  TreatAsAtomicUnit=on
  Permeate Flux Rate (L/min/m2) : Outport
  Permeate Salinity g/L : Outport  Port=2
  deltaPi_bar : Outport  Port=3
  wires:
  Salt Perm (L/m2/min)/1 -> MATLAB Function/5(B)
  <Feed Temperature (oC)>/1 -> MATLAB Function/1(T)
  <S1 Feed Salinity (g/L)>/1 -> MATLAB Function/6(cfeed)
  <S1 Feed Pressure (bar)>/1 -> MATLAB Function/2(Pfeed)
  cperm/1 -> MATLAB Function/7(cperm_prev)
  Pperm/1 -> MATLAB Function/3(Pperm)
  Jw/1 -> MATLAB Function/8(Jw_prev)
  Water Perm (L/m2/min/Bar)/1 -> MATLAB Function/4(A)
  dh/1 -> MATLAB Function/9(dh)
  L/1 -> MATLAB Function/10(L)
  u/1 -> MATLAB Function/11(u)
  MATLAB Function/1(Jw) -> Permeate Flux Rate (L/min/m2)/1  "Permeate Flux Rate (L/min/m2)"
  MATLAB Function/2(cperm) -> Permeate Salinity g/L/1  "PROS1_3_PermeateSalinity_gL"
  MATLAB Function/3(deltaPi_bar) -> deltaPi_bar/1

== system ARC_DTm/PROS1_4/Subsystem ==
  <Feed Temperature (oC)> : Inport
  <S1 Feed Pressure (bar)> : Inport  Port=2
  Pperm : Inport  Port=3
  Water Perm (L/m2/min/Bar) : Inport  Port=4
  Salt Perm (L/m2/min) : Inport  Port=5
  <S1 Feed Salinity (g/L)> : Inport  Port=6
  cperm : Inport  Port=7
  Jw : Inport  Port=8
  dh : Inport  Port=9
  L : Inport  Port=10
  u : Inport  Port=11
  MATLAB Function : MATLAB Function  TreatAsAtomicUnit=on
  Permeate Flux Rate (L/min/m2) : Outport
  Permeate Salinity g/L : Outport  Port=2
  deltaPi_bar : Outport  Port=3
  wires:
  Salt Perm (L/m2/min)/1 -> MATLAB Function/5(B)
  <Feed Temperature (oC)>/1 -> MATLAB Function/1(T)
  <S1 Feed Salinity (g/L)>/1 -> MATLAB Function/6(cfeed)
  <S1 Feed Pressure (bar)>/1 -> MATLAB Function/2(Pfeed)
  cperm/1 -> MATLAB Function/7(cperm_prev)
  Pperm/1 -> MATLAB Function/3(Pperm)
  Jw/1 -> MATLAB Function/8(Jw_prev)
  Water Perm (L/m2/min/Bar)/1 -> MATLAB Function/4(A)
  dh/1 -> MATLAB Function/9(dh)
  L/1 -> MATLAB Function/10(L)
  u/1 -> MATLAB Function/11(u)
  MATLAB Function/1(Jw) -> Permeate Flux Rate (L/min/m2)/1  "Permeate Flux Rate (L/min/m2)"
  MATLAB Function/2(cperm) -> Permeate Salinity g/L/1  "PROS1_4_PermeateSalinity_gL"
  MATLAB Function/3(deltaPi_bar) -> deltaPi_bar/1

== system ARC_DTm/PROS2_1/Subsystem ==
  <Feed Temperature (oC)> : Inport
  <S2 Feed Pressure (bar)> : Inport  Port=2
  Pperm : Inport  Port=3
  Water Perm (L/m2/min/Bar) : Inport  Port=4
  Salt Perm (L/m2/min) : Inport  Port=5
  <S2 Feed Salinity (g/L)> : Inport  Port=6
  cperm : Inport  Port=7
  Jw : Inport  Port=8
  dh : Inport  Port=9
  L : Inport  Port=10
  u : Inport  Port=11
  MATLAB Function : MATLAB Function  TreatAsAtomicUnit=on
  Permeate Flux Rate (L/min/m2) : Outport
  Permeate Salinity g/L : Outport  Port=2
  deltaPi_bar : Outport  Port=3
  wires:
  Salt Perm (L/m2/min)/1 -> MATLAB Function/5(B)
  <Feed Temperature (oC)>/1 -> MATLAB Function/1(T)
  <S2 Feed Salinity (g/L)>/1 -> MATLAB Function/6(cfeed)  "Feed Salinity g/L"
  <S2 Feed Pressure (bar)>/1 -> MATLAB Function/2(Pfeed)
  cperm/1 -> MATLAB Function/7(cperm_prev)
  Pperm/1 -> MATLAB Function/3(Pperm)
  Jw/1 -> MATLAB Function/8(Jw_prev)  "Permeate Flux (Jw)"
  Water Perm (L/m2/min/Bar)/1 -> MATLAB Function/4(A)
  dh/1 -> MATLAB Function/9(dh)
  L/1 -> MATLAB Function/10(L)
  u/1 -> MATLAB Function/11(u)  "Flow Velocity (cm/s)"
  MATLAB Function/1(Jw) -> Permeate Flux Rate (L/min/m2)/1  "Permeate Flux Rate (L/min/m2)"
  MATLAB Function/2(cperm) -> Permeate Salinity g/L/1  "PROS2_1_PermeateSalinity_gL"
  MATLAB Function/3(deltaPi_bar) -> deltaPi_bar/1

== system ARC_DTm/PROS2_2/Subsystem ==
  <Feed Temperature (oC)> : Inport
  <S2 Feed Pressure (bar)> : Inport  Port=2
  Pperm : Inport  Port=3
  Water Perm (L/m2/min/Bar) : Inport  Port=4
  Salt Perm (L/m2/min) : Inport  Port=5
  <S2 Feed Salinity (g/L)> : Inport  Port=6
  cperm : Inport  Port=7
  Jw : Inport  Port=8
  dh : Inport  Port=9
  L : Inport  Port=10
  u : Inport  Port=11
  MATLAB Function : MATLAB Function  TreatAsAtomicUnit=on
  Permeate Flux Rate (L/min/m2) : Outport
  Permeate Salinity g/L : Outport  Port=2
  deltaPi_bar : Outport  Port=3
  wires:
  Salt Perm (L/m2/min)/1 -> MATLAB Function/5(B)
  <Feed Temperature (oC)>/1 -> MATLAB Function/1(T)
  <S2 Feed Salinity (g/L)>/1 -> MATLAB Function/6(cfeed)  "Feed Salinity g/L"
  <S2 Feed Pressure (bar)>/1 -> MATLAB Function/2(Pfeed)
  cperm/1 -> MATLAB Function/7(cperm_prev)
  Pperm/1 -> MATLAB Function/3(Pperm)
  Jw/1 -> MATLAB Function/8(Jw_prev)  "Permeate Flux (Jw)"
  Water Perm (L/m2/min/Bar)/1 -> MATLAB Function/4(A)
  dh/1 -> MATLAB Function/9(dh)
  L/1 -> MATLAB Function/10(L)
  u/1 -> MATLAB Function/11(u)  "Flow Velocity (cm/s)"
  MATLAB Function/1(Jw) -> Permeate Flux Rate (L/min/m2)/1  "Permeate Flux Rate (L/min/m2)"
  MATLAB Function/2(cperm) -> Permeate Salinity g/L/1  "PROS2_2_PermeateSalinity_gL"
  MATLAB Function/3(deltaPi_bar) -> deltaPi_bar/1

== system ARC_DTm/PROS2_3/Subsystem ==
  <Feed Temperature (oC)> : Inport
  <S2 Feed Pressure (bar)> : Inport  Port=2
  Pperm : Inport  Port=3
  Water Perm (L/m2/min/Bar) : Inport  Port=4
  Salt Perm (L/m2/min) : Inport  Port=5
  <S2 Feed Salinity (g/L)> : Inport  Port=6
  cperm : Inport  Port=7
  Jw : Inport  Port=8
  dh : Inport  Port=9
  L : Inport  Port=10
  u : Inport  Port=11
  MATLAB Function : MATLAB Function  TreatAsAtomicUnit=on
  Permeate Flux Rate (L/min/m2) : Outport
  Permeate Salinity g/L : Outport  Port=2
  deltaPi_bar : Outport  Port=3
  wires:
  Salt Perm (L/m2/min)/1 -> MATLAB Function/5(B)
  <Feed Temperature (oC)>/1 -> MATLAB Function/1(T)
  <S2 Feed Salinity (g/L)>/1 -> MATLAB Function/6(cfeed)  "Feed Salinity g/L"
  <S2 Feed Pressure (bar)>/1 -> MATLAB Function/2(Pfeed)
  cperm/1 -> MATLAB Function/7(cperm_prev)
  Pperm/1 -> MATLAB Function/3(Pperm)
  Jw/1 -> MATLAB Function/8(Jw_prev)  "Permeate Flux (Jw)"
  Water Perm (L/m2/min/Bar)/1 -> MATLAB Function/4(A)
  dh/1 -> MATLAB Function/9(dh)
  L/1 -> MATLAB Function/10(L)
  u/1 -> MATLAB Function/11(u)  "Flow Velocity (cm/s)"
  MATLAB Function/1(Jw) -> Permeate Flux Rate (L/min/m2)/1  "Permeate Flux Rate (L/min/m2)"
  MATLAB Function/2(cperm) -> Permeate Salinity g/L/1  "PROS2_3_PermeateSalinity_gL"
  MATLAB Function/3(deltaPi_bar) -> deltaPi_bar/1

== system ARC_DTm/PROS2_4/Subsystem ==
  <Feed Temperature (oC)> : Inport
  <S2 Feed Pressure (bar)> : Inport  Port=2
  Pperm : Inport  Port=3
  Water Perm (L/m2/min/Bar) : Inport  Port=4
  Salt Perm (L/m2/min) : Inport  Port=5
  <S2 Feed Salinity (g/L)> : Inport  Port=6
  cperm : Inport  Port=7
  Jw : Inport  Port=8
  dh : Inport  Port=9
  L : Inport  Port=10
  u : Inport  Port=11
  MATLAB Function : MATLAB Function  TreatAsAtomicUnit=on
  Permeate Flux Rate (L/min/m2) : Outport
  Permeate Salinity g/L : Outport  Port=2
  deltaPi_bar : Outport  Port=3
  wires:
  Salt Perm (L/m2/min)/1 -> MATLAB Function/5(B)
  <Feed Temperature (oC)>/1 -> MATLAB Function/1(T)
  <S2 Feed Salinity (g/L)>/1 -> MATLAB Function/6(cfeed)  "Feed Salinity g/L"
  <S2 Feed Pressure (bar)>/1 -> MATLAB Function/2(Pfeed)
  cperm/1 -> MATLAB Function/7(cperm_prev)
  Pperm/1 -> MATLAB Function/3(Pperm)
  Jw/1 -> MATLAB Function/8(Jw_prev)  "Permeate Flux (Jw)"
  Water Perm (L/m2/min/Bar)/1 -> MATLAB Function/4(A)
  dh/1 -> MATLAB Function/9(dh)
  L/1 -> MATLAB Function/10(L)
  u/1 -> MATLAB Function/11(u)  "Flow Velocity (cm/s)"
  MATLAB Function/1(Jw) -> Permeate Flux Rate (L/min/m2)/1  "Permeate Flux Rate (L/min/m2)"
  MATLAB Function/2(cperm) -> Permeate Salinity g/L/1  "PROS2_4_PermeateSalinity_gL"
  MATLAB Function/3(deltaPi_bar) -> deltaPi_bar/1

== system ARC_DTm/Plant_LocalLoad_FMU/Battery System ==
  Solar In : Inport
  Local Load Demand : Inport  Port=2
  SOC : Inport  Port=3
  Basic Arbitrage : Subsystem  TreatAsAtomicUnit=on
  Battery Charge Setpoint : Merge  Inputs=3
  Battery Discharge Setpoint : Merge  Inputs=3
  Battery PID Solar Data : Subsystem  Commented=on
  Battery PID Solar Data1 : Subsystem  Commented=on
  Battery PID Solar Data2 : Subsystem  Commented=on
  Battery PID Solar Data3 : Subsystem  Commented=on
  Compare To Constant : simulink/Logic and Bit Operations/Compare To Constant  relop=<  const=3.9  OutDataTypeStr=boolean
  Compare To Constant1 : simulink/Logic and Bit Operations/Compare To Constant  relop=>  const=.1  OutDataTypeStr=boolean
  Constant : Constant  Value=batteryScenario
  Excess Solar : Subsystem  TreatAsAtomicUnit=on
  From{1..4} (4 alike) : From  Commented=on  GotoTag=SOC
  Gain : Gain  Commented=on  Gain=-1
  Goto : Goto  Commented=on  GotoTag=SOC
  If : If  IfExpression=u1 == 1  ElseIfExpressions=u1==2
  MWmin > MWh : Gain  Gain=1/60
  NoBattery : Subsystem  TreatAsAtomicUnit=on
  Product : Product
  Product1 : Product
  Scope : Scope  Commented=on  NumInputPorts=2
      settings: ActiveDisplayYMinimum=-1.0125  ActiveDisplayYMaximum=0.11249999999999998  DataLoggingVariableName=ScopeData5
  Scope1 : Scope  Commented=on  NumInputPorts=2
      settings: ActiveDisplayYMinimum=-0.96522618502196855  ActiveDisplayYMaximum=1.0322332055334107  DataLoggingVariableName=ScopeData6
  Scope2 : Scope  NumInputPorts=3
      settings: ActiveDisplayYMinimum=-0.24999999999999994  ActiveDisplayYMaximum=2.25  DataLoggingVariableName=ScopeData40
  Scope3 : Scope  NumInputPorts=2
      settings: ActiveDisplayYMinimum=-0.12499999999999997  ActiveDisplayYMaximum=1.125  DataLoggingVariableName=ScopeData41
  "Setpoint PID Solar+Battery " : Subsystem  Commented=on
  State-of-Charge (MWh) : Integrator  InitialCondition=2  LimitOutput=on  UpperSaturationLimit=3.9  LowerSaturationLimit=.1
  Sum : Sum  Inputs=+|-
  Unit Delay{1..4} (4 alike) : UnitDelay  Commented=on  SampleTime=-1  HasFrameUpgradeWarning=on
  Battery Charge : Outport
  Battery  discharge : Outport  Port=2
  wires:
  Unit Delay1/1 -> Battery PID Solar Data/2(feedback)
  From1/1 -> Unit Delay1/1
  "Setpoint PID Solar+Battery "/1(Setpoint BattCharge) -> Scope1/1, Battery PID Solar Data/1(Setpoint)
  Battery PID Solar Data/1(BatteryChargeDisch) -> Scope1/2
  "Setpoint PID Solar+Battery "/2(Setpoint BattDischarge) -> Scope/1, Battery PID Solar Data1/1(Setpoint)
  Battery PID Solar Data1/1(Battery Disch) -> Gain/1
  From2/1 -> Unit Delay2/1
  Unit Delay2/1 -> Battery PID Solar Data1/2(feedback)
  Gain/1 -> Scope/2
  Constant/1 -> If/1
  If/1 -> Excess Solar/Action
  Solar In/1 -> Excess Solar/1(Solar In)
  Local Load Demand/1 -> Excess Solar/2(Local Load Demand)
  If/2 -> Basic Arbitrage/Action
  If/3 -> NoBattery/Action
  Excess Solar/1(Battery Charge Command) -> Battery Charge Setpoint/1
  Basic Arbitrage/1(Battery Charge Command) -> Battery Charge Setpoint/2
  NoBattery/1(Battery Charge Request) -> Battery Charge Setpoint/3
  Excess Solar/2(Battery Discharge Command) -> Battery Discharge Setpoint/1
  Basic Arbitrage/2(Battery Discharge Command) -> Battery Discharge Setpoint/2
  NoBattery/2(Battery Discharge Request) -> Battery Discharge Setpoint/3
  Battery Charge Setpoint/1 -> Scope3/1, Sum/1, Product/1
  Product/1 -> Scope2/2, Battery Charge/1  "Battery Charge MW"
  Compare To Constant1/1 -> Product1/1
  SOC/1 -> [SOC]
  ? -> Battery PID Solar Data3/1(Setpoint)
  Unit Delay3/1 -> Battery PID Solar Data2/2(feedback)
  Unit Delay4/1 -> Battery PID Solar Data3/2(feedback)
  ? -> Battery PID Solar Data2/1(Setpoint)
  From4/1 -> Unit Delay4/1
  From3/1 -> Unit Delay3/1
  MWmin > MWh/1 -> State-of-Charge (MWh)/1
  Sum/1 -> MWmin > MWh/1
  Battery Discharge Setpoint/1 -> Scope3/2, Product1/2, Sum/2
  Compare To Constant/1 -> Product/2
  State-of-Charge (MWh)/1 -> Scope2/1, Compare To Constant/1, Compare To Constant1/1  "Battery SOC MWh"
  Product1/1 -> Scope2/3, Battery  discharge/1  "Battery Discharge MW"

== system ARC_DTm/Product Water Tank/Salinity Mass Balance ==
  InflowLoadingRate1 : Inport
  InflowLoadingRate2 : Inport  Port=2
  OutflowRate1 : Inport  Port=3
  OutflowRate2 : Inport  Port=4
  Volume (L3) : Inport  Port=5
  Mass Outflow (M/T) : Product
  Scope : Scope  NumInputPorts=2
      settings: Title=Raw Water Tank TSS  ActiveDisplayYMinimum=28.20057  ActiveDisplayYMaximum=44.64438  YLabel=Raw Water Tank TSS Concentration (ppm)
  Sum : Sum  Inputs=-++
  Sum1 : Sum  Inputs=++|
  Tank Concentration (CONC) : Integrator  InitialCondition=initTSS
  dc/dt (CONC/s) : Product  Inputs=*/
  TDS (CONC) : Outport
  wires:
  Sum1/1 -> Mass Outflow (M/T)/1  "Outflow Rate (FLOW)"
  Tank Concentration (CONC)/1 -> TDS (CONC)/1, Scope/1, Mass Outflow (M/T)/2  "TDS Concentration (CONC)"
  dc/dt (CONC/s)/1 -> Tank Concentration (CONC)/1
  Sum/1 -> dc/dt (CONC/s)/1
  Mass Outflow (M/T)/1 -> Scope/2, Sum/1  "Mass Outflow (LOADING)"
  InflowLoadingRate1/1 -> Sum/2  "M/T"
  InflowLoadingRate2/1 -> Sum/3
  OutflowRate1/1 -> Sum1/2  "L^3/T"
  OutflowRate2/1 -> Sum1/1  "L3/T"
  Volume (L3)/1 -> dc/dt (CONC/s)/2

== system ARC_DTm/Product Water Tank/TSS Mass Balance ==
  InflowLoadingRate1 : Inport
  InflowLoadingRate2 : Inport  Port=2
  OutflowRate1 : Inport  Port=3
  OutflowRate2 : Inport  Port=4
  Volume (L3) : Inport  Port=5
  Constant : Constant
  Mass Outflow (M/T) : Product
  Scope : Scope  NumInputPorts=2
      settings: Title=Raw Water Tank TSS  ActiveDisplayYMinimum=41.63707  ActiveDisplayYMaximum=43.15144  YLabel=Raw Water Tank TSS Concentration (ppm)
  Scope1 : Scope
  Sum : Sum  Inputs=-++
  Sum1 : Sum  Inputs=++|
  Tank Concentration (CONC) : Integrator  InitialCondition=initTSS
  TSS Concentration (CONC) : Outport
  wires:
  Sum1/1 -> Mass Outflow (M/T)/1  "Outflow Rate (FLOW)"
  Tank Concentration (CONC)/1 -> Scope1/1, TSS Concentration (CONC)/1, Mass Outflow (M/T)/2, Scope/1  "TSS Concentration (CONC)"
  Constant/1 -> Tank Concentration (CONC)/1
  Sum/1 -> ?
  Mass Outflow (M/T)/1 -> Scope/2, Sum/1  "Mass Outflow (LOADING)"
  InflowLoadingRate1/1 -> Sum/2  "M/T"
  InflowLoadingRate2/1 -> Sum/3
  OutflowRate1/1 -> Sum1/2  "L^3/T"
  OutflowRate2/1 -> Sum1/1  "L3/T"
  Volume (L3)/1 -> ?

== system ARC_DTm/Product Water Tank/Tank Storage ==
  <Flow Rate (FLOW)> : Inport
  <Permeate Flow (FLOW)> : Inport  Port=2
  <Pump Flow (FLOW)> : Inport  Port=3
  Inflow Rate : Sum
  Lower Operating Limit : Gain  Gain=volMin
  Manage Overflows : Subsystem
      settings: PortSchema="{\"entries\":[{\"content\":{\"sides\":[{\"content\":{\"connectorIds\":[\"In1\",\"In2\",\"In3\"]},\"type\":\"ConnectorPlacement.EquallySpacedRectSide\",\"uuid\":\"13451602-39ff-4826-b8b0-c0861768c7fb\"},{\"content\":{\"connectorIds\":[\"Out1\",\"Out2\",\"Out3\",\"Out4\"],\"side\":\"RIGHT\"},\"type\":\"ConnectorPlacement.EquallySpacedRectSide\",\"uuid\":\"b2aad888-ad49-48b8-8c51-33a8557894eb\"},{\"content\":{\"side\":\"TOP\"},\"type\":\"ConnectorPlacement.EquallySpacedRectSide\",\"uuid\":\"da6eb0b1-b17a-44e2-9b47-47b80b3dfaff\"},{\"content\":{\"connectorIds\":[\"In4\"],\"side\":\"BOTTOM\"},\"type\":\"ConnectorPlacement.EquallySpacedRectSide\",\"uuid\":\"0d27dbd4-d10f-4713-b2f6-efd1be865b8f\"}]},\"type\":\"ConnectorPlacement.EquallySpacedConnector\",\"uuid\":\"58d86696-4d30-4c65-b93d-3b184314107e\"}],\"packageUris\":[\"http://schema.mathworks.com/mf0/Connector/R2020b\"],\"version\":\"1.0\"}"
  Memory : Memory  LinearizeAsDelay=on
  Net Flow : Sum  Inputs=|+-
  New Tank Volume: V(t) [VOL] : Integrator  InitialCondition=initVol * vol
  Scope : Scope  NumInputPorts=3
      settings: ActiveDisplayYMinimum=-4.26687  ActiveDisplayYMaximum=88.40187
  Scope1 : Scope  NumInputPorts=3
      settings: ActiveDisplayYMinimum=93.75  ActiveDisplayYMaximum=406.25  DataLoggingVariableName=ScopeData4
  Tank Volume (VOL) : Constant  Value=vol
  Upper Operating Limit : Gain  Gain=volMax
  VolumeConditions : Subsystem
  Well Flow Rate (FLOW) : Outport
  RO Perm Flow Rate (FLOW) : Outport  Port=2
  Pump Flow Rate (FLOW) : Outport  Port=3
  Volume (VOL) : Outport  Port=4
  wires:
  <Flow Rate (FLOW)>/1 -> Manage Overflows/2(<Flow Rate (FLOW)>)
  <Pump Flow (FLOW)>/1 -> Manage Overflows/4(Pump Flow (FLOW))
  <Permeate Flow (FLOW)>/1 -> Manage Overflows/3(<Permeate Flow (FLOW)>)
  Net Flow/1 -> New Tank Volume: V(t) [VOL]/1  "dV/dt (FLOW)"
  Manage Overflows/3(Pump Flow Rate (FLOW)) -> Net Flow/2, Pump Flow Rate (FLOW)/1, Scope/3  "Pump Flow Rate (FLOW)"
  Inflow Rate/1 -> Net Flow/1
  Manage Overflows/2(RO Perm Flow Rate (FLOW)) -> Inflow Rate/2, RO Perm Flow Rate (FLOW)/1, Scope/2  "RO Perm Flow Rate (FLOW)"
  Manage Overflows/1(Well Flow Rate (FLOW)) -> Inflow Rate/1, Well Flow Rate (FLOW)/1, Scope/1  "Well Flow Rate (FLOW)"
  New Tank Volume: V(t) [VOL]/1 -> Scope1/1, VolumeConditions/1(Stored Volume (VOL)), Volume (VOL)/1  "FLOW"
  Tank Volume (VOL)/1 -> Upper Operating Limit/1, Lower Operating Limit/1, VolumeConditions/2(Tank Volume (VOL))
  VolumeConditions/1(Cooldown Timer) -> Manage Overflows/1(Timer)
  Upper Operating Limit/1 -> Scope1/2
  Lower Operating Limit/1 -> Scope1/3
  Manage Overflows/4(TimerOut) -> Memory/1
  Memory/1 -> VolumeConditions/3(Timer)
